simulink model "flanger_ref"  (R2020b)
settings: Solver=FixedStepDiscrete  StartTime=0.0  StopTime=stopTime  FixedStep=1.0416666666666666e-05  RelTol=1e-3
settings Model: Creator=Ross  LastModifiedBy=wickh
settings DataIOCC: SaveOutput=off  SaveTime=off  ReturnWorkspaceOutputs=off
settings OptimizationCC: BlockReduction=off  ConditionallyExecuteInputs=off  DefaultParameterBehavior=Inlined  SimCompilerOptimization=on
settings DebuggingCC: ReadBeforeWriteMsg=DisableAll  WriteAfterWriteMsg=DisableAll  WriteAfterReadMsg=DisableAll  AlgebraicLoopMsg=error  MultiTaskDSMMsg=none  SingleTaskRateTransMsg=error  PregeneratedLibrarySubsystemCodeDiagnostic=none  ArithmeticOperatorsInVariantConditions=warning
settings HardwareCC: ProdBitPerPointer=32  ProdBitPerSizeT=32  ProdBitPerPtrDiffT=32  ProdLargestAtomicFloat=None  ProdIntDivRoundTo=Undefined  ProdEndianess=Unspecified  ProdWordSize=32  ProdHWDeviceType=ASIC/FPGA->ASIC/FPGA  TargetBitPerPointer=64  TargetBitPerSizeT=64  TargetBitPerPtrDiffT=64  TargetLongLongMode=on  TargetIntDivRoundTo=Zero  TargetEndianess=LittleEndian  TargetWordSize=64  TargetHWDeviceType=Custom Processor->MATLAB Host Computer  ProdEqTarget=off
settings ModelReferenceCC: UpdateModelReferenceTargets=IfOutOfDate
settings SFSimCC: SFSimEcho=off  SimUseLocalCustomCode=off  CustomCodeUndefinedFunction=UseInterfaceOnly
settings RTWCC: RTWUseLocalCustomCode=off

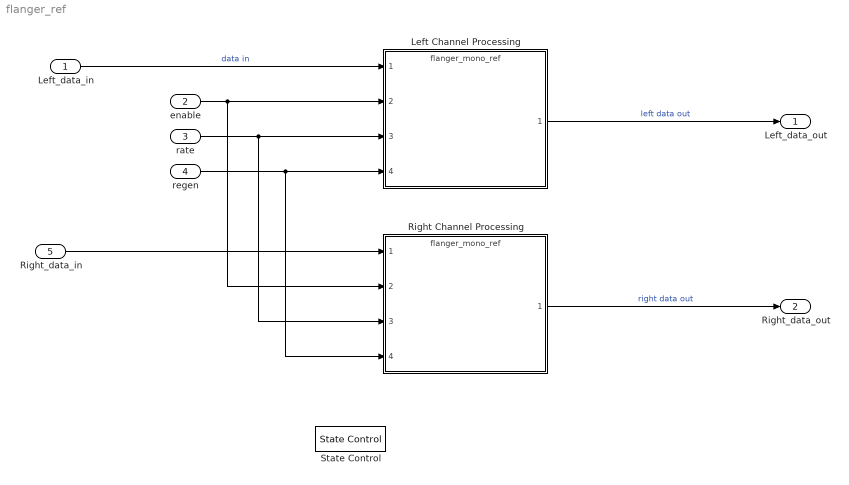
== system flanger_ref ==
  Left_data_in : Inport  OutDataTypeStr=fixdt(1,24,23)  PortDimensions=1
  enable : Inport  Port=2  OutDataTypeStr=boolean  PortDimensions=1
  rate : Inport  Port=3  OutDataTypeStr=rate_dt  PortDimensions=1
  regen : Inport  Port=4  OutDataTypeStr=regen_dt  PortDimensions=1
  Right_data_in : Inport  Port=5  OutDataTypeStr=fixdt(1,24,23)  PortDimensions=1
  Left Channel Processing : ModelReference  ModelNameDialog=flanger_mono_ref  SimulationMode=Normal  ModelReferenceVersion=3.18
  Right Channel Processing : ModelReference  ModelNameDialog=flanger_mono_ref  SimulationMode=Normal  ModelReferenceVersion=3.18
  State Control : StateControl  StateControl=Synchronous
  Left_data_out : Outport  OutDataTypeStr=fixdt(1,24,23)  PortDimensions=1  InitialOutput=0  VectorParamsAs1DForOutWhenUnconnected=off
  Right_data_out : Outport  Port=2  OutDataTypeStr=fixdt(1,24,23)  PortDimensions=1
  wires:
  rate/1 -> Left Channel Processing/3, Right Channel Processing/3
  regen/1 -> Left Channel Processing/4, Right Channel Processing/4
  enable/1 -> Left Channel Processing/2, Right Channel Processing/2
  Left_data_in/1 -> Left Channel Processing/1  "data in"
  Right_data_in/1 -> Right Channel Processing/1
  Left Channel Processing/1 -> Left_data_out/1  "left data out"
  Right Channel Processing/1 -> Right_data_out/1  "right data out"
